simulink model "jplsetispec_thresh_rev003"  (Simulink 6.2)
settings: Solver=ode45  StartTime=0.0  StopTime=100  RelTol=1e-3
libraries: xbsIndex_r3 x776, xps_library x53, casper_library x4
(part 2 of 5)

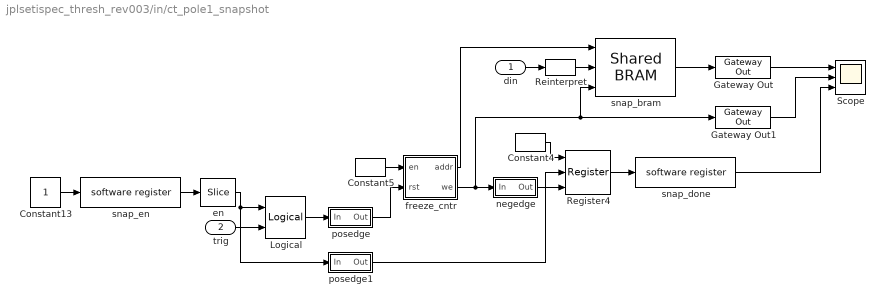
== system jplsetispec_thresh_rev003/in/ct_pole1_snapshot ==
  din : Inport  Port=1  LatchInput=off
  trig : Inport  Port=2  LatchInput=off
  Constant13 : Constant
  Constant4 : xbsIndex_r3/Constant  const=1  equ=P=C  arith_type=Unsigned  n_bits=1  bin_pt=0  opselect=C  inp2=PCIN>>17  opr=+  inp1=P  carry=CIN  iostate=0  explicit_period=on  period=1  dbl_ovrd=off
  Constant5 : xbsIndex_r3/Constant  const=1  equ=P=C  arith_type=Boolean  n_bits=1  bin_pt=0  opselect=C  inp2=PCIN>>17  opr=+  inp1=P  carry=CIN  iostate=0  explicit_period=on  period=1  dbl_ovrd=off
  Gateway Out : xbsIndex_r3/Gateway Out  output_type=Double  nbits=8  bin_pt=6  arith_type=Boolean  quantization=Truncate  overflow=Wrap  hdl_port=off  timing_constraint=None  locs_specified=off  LOCs={}  needs_fixed_name=off  show_param=off
      settings: xl_area=[0, 0, 0, 0, 0, 0, 0]
  Gateway Out1 : xbsIndex_r3/Gateway Out  output_type=Double  nbits=8  bin_pt=6  arith_type=Boolean  quantization=Truncate  overflow=Wrap  hdl_port=off  timing_constraint=None  locs_specified=off  LOCs={}  needs_fixed_name=off  show_param=off
      settings: xl_area=[0, 0, 0, 0, 0, 0, 0]
  Logical : xbsIndex_r3/Logical  logical_function=AND  inputs=2  precision=Full  arith_type=Unsigned  n_bits=8  bin_pt=2  align_bp=on  latency=0  explicit_period=on  period=1  en=off  dbl_ovrd=off  show_param=off
      settings: xl_area=[0, 0, 0, 0, 0, 0, 0]
  Register4 : xbsIndex_r3/Register  init=0  reg_only_valid=off  explicit_period=off  period=1  rst=on  en=on  out_en=off  dbl_ovrd=off  show_param=off
      settings: xl_area=[0, 0, 0, 0, 0, 0, 0]
  Reinterpret : xbsIndex_r3/Reinterpret  force_arith_type=on  arith_type=Unsigned  force_bin_pt=on  bin_pt=0  force_valid=on
  Scope : Scope  NumInputPorts=3
      settings: YMin=-5~-5~-5  YMax=5~5~5
  en : xbsIndex_r3/Slice  mode=Lower Bit Location + Width  nbits=1  bit1=0  base1=LSB of Input  bit0=0  base0=LSB of Input  boolean_output=on  explicit_period=off  period=1  dbl_ovrd=off
  freeze_cntr : Subsystem  mask{CounterBits=nsamples}
      mask prompts: CounterBits "Counter Length (2^?)"
  negedge : Subsystem  Tag=Rising Edge Detector
  posedge : Subsystem  Tag=Rising Edge Detector
  posedge1 : Subsystem  Tag=Rising Edge Detector
  snap_bram : xps_library/Shared BRAM  Tag=xps:bram  arith_type=Unsigned  addr_width=nsamples  data_width=32  data_bin_pt=0  init_vals=0  sample_rate=1
  snap_done : xps_library/software register  Tag=xps:sw_reg  io_dir=To Processor  arith_type=Unsigned  bitwidth=32  bin_pt=0  sample_period=1  gw_name=jplsetispec_thresh_rev003_in_ct_pole1_snapshot_snap_done_user_data_in
  snap_en : xps_library/software register  Tag=xps:sw_reg  io_dir=From Processor  arith_type=Unsigned  bitwidth=32  bin_pt=0  sample_period=1  gw_name=jplsetispec_thresh_rev003_in_ct_pole1_snapshot_snap_en_user_data_out
  wires:
  posedge1/1(Out) -> Register4/2
  snap_done/1 -> Scope/3
  Gateway Out1/1 -> Scope/2
  Gateway Out/1 -> Scope/1
  snap_bram/1 -> Gateway Out/1
  freeze_cntr/1(addr) -> snap_bram/1
  en/1 -> posedge1/1(In), Logical/1
  negedge/1(Out) -> Register4/3
  trig/1 -> Logical/2
  posedge/1(Out) -> freeze_cntr/2(rst)
  Logical/1 -> posedge/1(In)
  freeze_cntr/2(we) -> Gateway Out1/1, snap_bram/3, negedge/1(In)
  Constant5/1 -> freeze_cntr/1(en)
  Constant4/1 -> Register4/1
  Register4/1 -> snap_done/1
  Constant13/1 -> snap_en/1
  Reinterpret/1 -> snap_bram/2
  din/1 -> Reinterpret/1
  snap_en/1 -> en/1

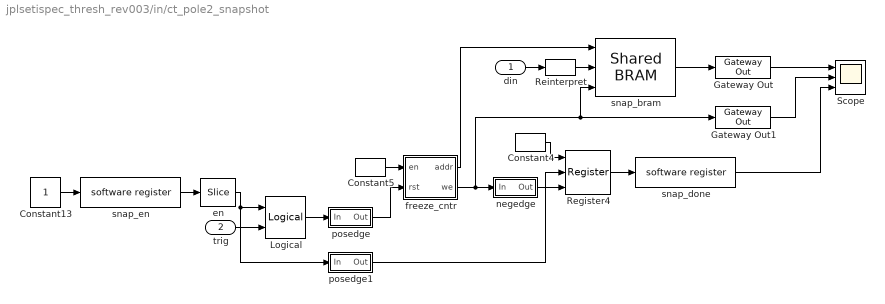
== system jplsetispec_thresh_rev003/in/ct_pole2_snapshot ==
  din : Inport  Port=1  LatchInput=off
  trig : Inport  Port=2  LatchInput=off
  Constant13 : Constant
  Constant4 : xbsIndex_r3/Constant  const=1  equ=P=C  arith_type=Unsigned  n_bits=1  bin_pt=0  opselect=C  inp2=PCIN>>17  opr=+  inp1=P  carry=CIN  iostate=0  explicit_period=on  period=1  dbl_ovrd=off
  Constant5 : xbsIndex_r3/Constant  const=1  equ=P=C  arith_type=Boolean  n_bits=1  bin_pt=0  opselect=C  inp2=PCIN>>17  opr=+  inp1=P  carry=CIN  iostate=0  explicit_period=on  period=1  dbl_ovrd=off
  Gateway Out : xbsIndex_r3/Gateway Out  output_type=Double  nbits=8  bin_pt=6  arith_type=Boolean  quantization=Truncate  overflow=Wrap  hdl_port=off  timing_constraint=None  locs_specified=off  LOCs={}  needs_fixed_name=off  show_param=off
      settings: xl_area=[0, 0, 0, 0, 0, 0, 0]
  Gateway Out1 : xbsIndex_r3/Gateway Out  output_type=Double  nbits=8  bin_pt=6  arith_type=Boolean  quantization=Truncate  overflow=Wrap  hdl_port=off  timing_constraint=None  locs_specified=off  LOCs={}  needs_fixed_name=off  show_param=off
      settings: xl_area=[0, 0, 0, 0, 0, 0, 0]
  Logical : xbsIndex_r3/Logical  logical_function=AND  inputs=2  precision=Full  arith_type=Unsigned  n_bits=8  bin_pt=2  align_bp=on  latency=0  explicit_period=on  period=1  en=off  dbl_ovrd=off  show_param=off
      settings: xl_area=[0, 0, 0, 0, 0, 0, 0]
  Register4 : xbsIndex_r3/Register  init=0  reg_only_valid=off  explicit_period=off  period=1  rst=on  en=on  out_en=off  dbl_ovrd=off  show_param=off
      settings: xl_area=[0, 0, 0, 0, 0, 0, 0]
  Reinterpret : xbsIndex_r3/Reinterpret  force_arith_type=on  arith_type=Unsigned  force_bin_pt=on  bin_pt=0  force_valid=on
  Scope : Scope  NumInputPorts=3
      settings: YMin=-5~-5~-5  YMax=5~5~5
  en : xbsIndex_r3/Slice  mode=Lower Bit Location + Width  nbits=1  bit1=0  base1=LSB of Input  bit0=0  base0=LSB of Input  boolean_output=on  explicit_period=off  period=1  dbl_ovrd=off
  freeze_cntr : Subsystem  mask{CounterBits=nsamples}
      mask prompts: CounterBits "Counter Length (2^?)"
  negedge : Subsystem  Tag=Rising Edge Detector
  posedge : Subsystem  Tag=Rising Edge Detector
  posedge1 : Subsystem  Tag=Rising Edge Detector
  snap_bram : xps_library/Shared BRAM  Tag=xps:bram  arith_type=Unsigned  addr_width=nsamples  data_width=32  data_bin_pt=0  init_vals=0  sample_rate=1
  snap_done : xps_library/software register  Tag=xps:sw_reg  io_dir=To Processor  arith_type=Unsigned  bitwidth=32  bin_pt=0  sample_period=1  gw_name=jplsetispec_thresh_rev003_in_ct_pole2_snapshot_snap_done_user_data_in
  snap_en : xps_library/software register  Tag=xps:sw_reg  io_dir=From Processor  arith_type=Unsigned  bitwidth=32  bin_pt=0  sample_period=1  gw_name=jplsetispec_thresh_rev003_in_ct_pole2_snapshot_snap_en_user_data_out
  wires:
  snap_en/1 -> en/1
  din/1 -> Reinterpret/1
  Reinterpret/1 -> snap_bram/2
  Constant13/1 -> snap_en/1
  Register4/1 -> snap_done/1
  Constant4/1 -> Register4/1
  Constant5/1 -> freeze_cntr/1(en)
  freeze_cntr/2(we) -> negedge/1(In), snap_bram/3, Gateway Out1/1
  Logical/1 -> posedge/1(In)
  posedge/1(Out) -> freeze_cntr/2(rst)
  trig/1 -> Logical/2
  negedge/1(Out) -> Register4/3
  en/1 -> Logical/1, posedge1/1(In)
  freeze_cntr/1(addr) -> snap_bram/1
  snap_bram/1 -> Gateway Out/1
  Gateway Out/1 -> Scope/1
  Gateway Out1/1 -> Scope/2
  snap_done/1 -> Scope/3
  posedge1/1(Out) -> Register4/2

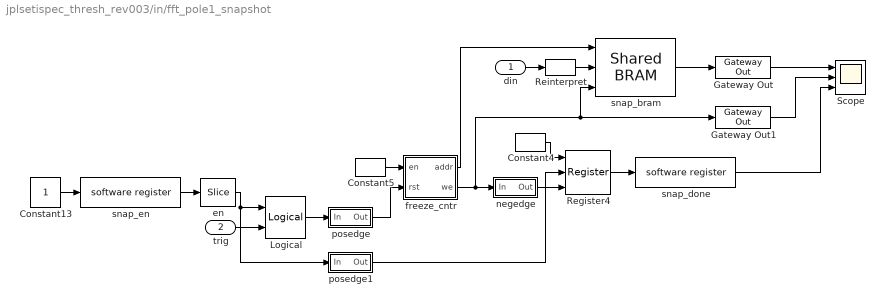
== system jplsetispec_thresh_rev003/in/fft_pole1_snapshot ==
  din : Inport  Port=1  LatchInput=off
  trig : Inport  Port=2  LatchInput=off
  Constant13 : Constant
  Constant4 : xbsIndex_r3/Constant  const=1  equ=P=C  arith_type=Unsigned  n_bits=1  bin_pt=0  opselect=C  inp2=PCIN>>17  opr=+  inp1=P  carry=CIN  iostate=0  explicit_period=on  period=1  dbl_ovrd=off
  Constant5 : xbsIndex_r3/Constant  const=1  equ=P=C  arith_type=Boolean  n_bits=1  bin_pt=0  opselect=C  inp2=PCIN>>17  opr=+  inp1=P  carry=CIN  iostate=0  explicit_period=on  period=1  dbl_ovrd=off
  Gateway Out : xbsIndex_r3/Gateway Out  output_type=Double  nbits=8  bin_pt=6  arith_type=Boolean  quantization=Truncate  overflow=Wrap  hdl_port=off  timing_constraint=None  locs_specified=off  LOCs={}  needs_fixed_name=off  show_param=off
      settings: xl_area=[0, 0, 0, 0, 0, 0, 0]
  Gateway Out1 : xbsIndex_r3/Gateway Out  output_type=Double  nbits=8  bin_pt=6  arith_type=Boolean  quantization=Truncate  overflow=Wrap  hdl_port=off  timing_constraint=None  locs_specified=off  LOCs={}  needs_fixed_name=off  show_param=off
      settings: xl_area=[0, 0, 0, 0, 0, 0, 0]
  Logical : xbsIndex_r3/Logical  logical_function=AND  inputs=2  precision=Full  arith_type=Unsigned  n_bits=8  bin_pt=2  align_bp=on  latency=0  explicit_period=on  period=1  en=off  dbl_ovrd=off  show_param=off
      settings: xl_area=[0, 0, 0, 0, 0, 0, 0]
  Register4 : xbsIndex_r3/Register  init=0  reg_only_valid=off  explicit_period=off  period=1  rst=on  en=on  out_en=off  dbl_ovrd=off  show_param=off
      settings: xl_area=[0, 0, 0, 0, 0, 0, 0]
  Reinterpret : xbsIndex_r3/Reinterpret  force_arith_type=on  arith_type=Unsigned  force_bin_pt=on  bin_pt=0  force_valid=on
  Scope : Scope  NumInputPorts=3
      settings: YMin=-5~-5~-5  YMax=5~5~5
  en : xbsIndex_r3/Slice  mode=Lower Bit Location + Width  nbits=1  bit1=0  base1=LSB of Input  bit0=0  base0=LSB of Input  boolean_output=on  explicit_period=off  period=1  dbl_ovrd=off
  freeze_cntr : Subsystem  mask{CounterBits=nsamples}
      mask prompts: CounterBits "Counter Length (2^?)"
  negedge : Subsystem  Tag=Rising Edge Detector
  posedge : Subsystem  Tag=Rising Edge Detector
  posedge1 : Subsystem  Tag=Rising Edge Detector
  snap_bram : xps_library/Shared BRAM  Tag=xps:bram  arith_type=Unsigned  addr_width=nsamples  data_width=32  data_bin_pt=0  init_vals=0  sample_rate=1
  snap_done : xps_library/software register  Tag=xps:sw_reg  io_dir=To Processor  arith_type=Unsigned  bitwidth=32  bin_pt=0  sample_period=1  gw_name=jplsetispec_thresh_rev003_in_fft_pole1_snapshot_snap_done_user_data_in
  snap_en : xps_library/software register  Tag=xps:sw_reg  io_dir=From Processor  arith_type=Unsigned  bitwidth=32  bin_pt=0  sample_period=1  gw_name=jplsetispec_thresh_rev003_in_fft_pole1_snapshot_snap_en_user_data_out
  wires:
  posedge1/1(Out) -> Register4/2
  snap_done/1 -> Scope/3
  Gateway Out1/1 -> Scope/2
  Gateway Out/1 -> Scope/1
  snap_bram/1 -> Gateway Out/1
  freeze_cntr/1(addr) -> snap_bram/1
  en/1 -> posedge1/1(In), Logical/1
  negedge/1(Out) -> Register4/3
  trig/1 -> Logical/2
  posedge/1(Out) -> freeze_cntr/2(rst)
  Logical/1 -> posedge/1(In)
  freeze_cntr/2(we) -> Gateway Out1/1, snap_bram/3, negedge/1(In)
  Constant5/1 -> freeze_cntr/1(en)
  Constant4/1 -> Register4/1
  Register4/1 -> snap_done/1
  Constant13/1 -> snap_en/1
  Reinterpret/1 -> snap_bram/2
  din/1 -> Reinterpret/1
  snap_en/1 -> en/1

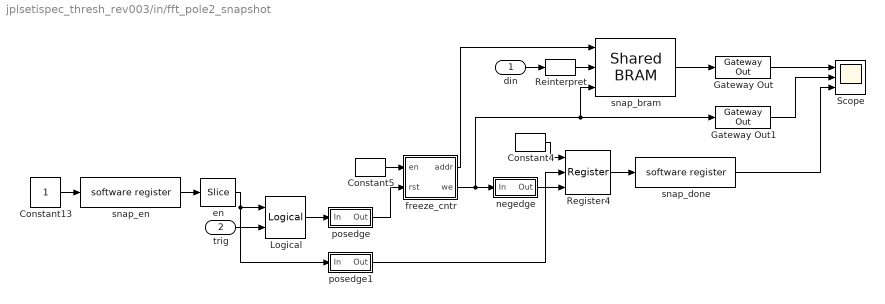
== system jplsetispec_thresh_rev003/in/fft_pole2_snapshot ==
  din : Inport  Port=1  LatchInput=off
  trig : Inport  Port=2  LatchInput=off
  Constant13 : Constant
  Constant4 : xbsIndex_r3/Constant  const=1  equ=P=C  arith_type=Unsigned  n_bits=1  bin_pt=0  opselect=C  inp2=PCIN>>17  opr=+  inp1=P  carry=CIN  iostate=0  explicit_period=on  period=1  dbl_ovrd=off
  Constant5 : xbsIndex_r3/Constant  const=1  equ=P=C  arith_type=Boolean  n_bits=1  bin_pt=0  opselect=C  inp2=PCIN>>17  opr=+  inp1=P  carry=CIN  iostate=0  explicit_period=on  period=1  dbl_ovrd=off
  Gateway Out : xbsIndex_r3/Gateway Out  output_type=Double  nbits=8  bin_pt=6  arith_type=Boolean  quantization=Truncate  overflow=Wrap  hdl_port=off  timing_constraint=None  locs_specified=off  LOCs={}  needs_fixed_name=off  show_param=off
      settings: xl_area=[0, 0, 0, 0, 0, 0, 0]
  Gateway Out1 : xbsIndex_r3/Gateway Out  output_type=Double  nbits=8  bin_pt=6  arith_type=Boolean  quantization=Truncate  overflow=Wrap  hdl_port=off  timing_constraint=None  locs_specified=off  LOCs={}  needs_fixed_name=off  show_param=off
      settings: xl_area=[0, 0, 0, 0, 0, 0, 0]
  Logical : xbsIndex_r3/Logical  logical_function=AND  inputs=2  precision=Full  arith_type=Unsigned  n_bits=8  bin_pt=2  align_bp=on  latency=0  explicit_period=on  period=1  en=off  dbl_ovrd=off  show_param=off
      settings: xl_area=[0, 0, 0, 0, 0, 0, 0]
  Register4 : xbsIndex_r3/Register  init=0  reg_only_valid=off  explicit_period=off  period=1  rst=on  en=on  out_en=off  dbl_ovrd=off  show_param=off
      settings: xl_area=[0, 0, 0, 0, 0, 0, 0]
  Reinterpret : xbsIndex_r3/Reinterpret  force_arith_type=on  arith_type=Unsigned  force_bin_pt=on  bin_pt=0  force_valid=on
  Scope : Scope  NumInputPorts=3
      settings: YMin=-5~-5~-5  YMax=5~5~5
  en : xbsIndex_r3/Slice  mode=Lower Bit Location + Width  nbits=1  bit1=0  base1=LSB of Input  bit0=0  base0=LSB of Input  boolean_output=on  explicit_period=off  period=1  dbl_ovrd=off
  freeze_cntr : Subsystem  mask{CounterBits=nsamples}
      mask prompts: CounterBits "Counter Length (2^?)"
  negedge : Subsystem  Tag=Rising Edge Detector
  posedge : Subsystem  Tag=Rising Edge Detector
  posedge1 : Subsystem  Tag=Rising Edge Detector
  snap_bram : xps_library/Shared BRAM  Tag=xps:bram  arith_type=Unsigned  addr_width=nsamples  data_width=32  data_bin_pt=0  init_vals=0  sample_rate=1
  snap_done : xps_library/software register  Tag=xps:sw_reg  io_dir=To Processor  arith_type=Unsigned  bitwidth=32  bin_pt=0  sample_period=1  gw_name=jplsetispec_thresh_rev003_in_fft_pole2_snapshot_snap_done_user_data_in
  snap_en : xps_library/software register  Tag=xps:sw_reg  io_dir=From Processor  arith_type=Unsigned  bitwidth=32  bin_pt=0  sample_period=1  gw_name=jplsetispec_thresh_rev003_in_fft_pole2_snapshot_snap_en_user_data_out
  wires:
  snap_en/1 -> en/1
  din/1 -> Reinterpret/1
  Reinterpret/1 -> snap_bram/2
  Constant13/1 -> snap_en/1
  Register4/1 -> snap_done/1
  Constant4/1 -> Register4/1
  Constant5/1 -> freeze_cntr/1(en)
  freeze_cntr/2(we) -> negedge/1(In), snap_bram/3, Gateway Out1/1
  Logical/1 -> posedge/1(In)
  posedge/1(Out) -> freeze_cntr/2(rst)
  trig/1 -> Logical/2
  negedge/1(Out) -> Register4/3
  en/1 -> Logical/1, posedge1/1(In)
  freeze_cntr/1(addr) -> snap_bram/1
  snap_bram/1 -> Gateway Out/1
  Gateway Out/1 -> Scope/1
  Gateway Out1/1 -> Scope/2
  snap_done/1 -> Scope/3
  posedge1/1(Out) -> Register4/2

== system jplsetispec_thresh_rev003/in/posedge ==
  in : Inport  Port=1  LatchInput=off
  Delay : xbsIndex_r3/Delay  latency=1  reg_retiming=off  explicit_period=off  period=1  en=off  accept_only_valid=off  init_zero=on  dbl_ovrd=off  show_param=off
      settings: xl_area=[0, 0, 0, 0, 0, 0, 0]
  Inverter : xbsIndex_r3/Inverter  latency=0  explicit_period=off  period=1  en=off  dbl_ovrd=off  show_param=off
      settings: xl_area=[0, 0, 0, 0, 0, 0, 0]
  Logical : xbsIndex_r3/Logical  logical_function=AND  inputs=2  precision=Full  arith_type=Unsigned  n_bits=8  bin_pt=2  align_bp=on  latency=0  explicit_period=off  period=1  en=off  dbl_ovrd=off  show_param=off
      settings: xl_area=[0, 0, 0, 0, 0, 0, 0]
  detect : Outport
  wires:
  Logical/1 -> detect/1
  in/1 -> Logical/2, Delay/1
  Inverter/1 -> Logical/1
  Delay/1 -> Inverter/1

== system jplsetispec_thresh_rev003/in/posedge1 ==
  in : Inport  Port=1  LatchInput=off
  Delay : xbsIndex_r3/Delay  latency=1  reg_retiming=off  explicit_period=off  period=1  en=off  accept_only_valid=off  init_zero=on  dbl_ovrd=off  show_param=off
      settings: xl_area=[0, 0, 0, 0, 0, 0, 0]
  Inverter : xbsIndex_r3/Inverter  latency=0  explicit_period=off  period=1  en=off  dbl_ovrd=off  show_param=off
      settings: xl_area=[0, 0, 0, 0, 0, 0, 0]
  Logical : xbsIndex_r3/Logical  logical_function=AND  inputs=2  precision=Full  arith_type=Unsigned  n_bits=8  bin_pt=2  align_bp=on  latency=0  explicit_period=off  period=1  en=off  dbl_ovrd=off  show_param=off
      settings: xl_area=[0, 0, 0, 0, 0, 0, 0]
  detect : Outport
  wires:
  Delay/1 -> Inverter/1
  Inverter/1 -> Logical/1
  in/1 -> Delay/1, Logical/2
  Logical/1 -> detect/1

== system jplsetispec_thresh_rev003/in/posedge2 ==
  in : Inport  Port=1  LatchInput=off
  Delay : xbsIndex_r3/Delay  latency=1  reg_retiming=off  explicit_period=off  period=1  en=off  accept_only_valid=off  init_zero=on  dbl_ovrd=off  show_param=off
      settings: xl_area=[0, 0, 0, 0, 0, 0, 0]
  Inverter : xbsIndex_r3/Inverter  latency=0  explicit_period=off  period=1  en=off  dbl_ovrd=off  show_param=off
      settings: xl_area=[0, 0, 0, 0, 0, 0, 0]
  Logical : xbsIndex_r3/Logical  logical_function=AND  inputs=2  precision=Full  arith_type=Unsigned  n_bits=8  bin_pt=2  align_bp=on  latency=0  explicit_period=off  period=1  en=off  dbl_ovrd=off  show_param=off
      settings: xl_area=[0, 0, 0, 0, 0, 0, 0]
  detect : Outport
  wires:
  Delay/1 -> Inverter/1
  Inverter/1 -> Logical/1
  in/1 -> Delay/1, Logical/2
  Logical/1 -> detect/1

== system jplsetispec_thresh_rev003/in/posedge3 ==
  in : Inport  Port=1  LatchInput=off
  Delay : xbsIndex_r3/Delay  latency=1  reg_retiming=off  explicit_period=off  period=1  en=off  accept_only_valid=off  init_zero=on  dbl_ovrd=off  show_param=off
      settings: xl_area=[0, 0, 0, 0, 0, 0, 0]
  Inverter : xbsIndex_r3/Inverter  latency=0  explicit_period=off  period=1  en=off  dbl_ovrd=off  show_param=off
      settings: xl_area=[0, 0, 0, 0, 0, 0, 0]
  Logical : xbsIndex_r3/Logical  logical_function=AND  inputs=2  precision=Full  arith_type=Unsigned  n_bits=8  bin_pt=2  align_bp=on  latency=0  explicit_period=off  period=1  en=off  dbl_ovrd=off  show_param=off
      settings: xl_area=[0, 0, 0, 0, 0, 0, 0]
  detect : Outport
  wires:
  Logical/1 -> detect/1
  in/1 -> Logical/2, Delay/1
  Inverter/1 -> Logical/1
  Delay/1 -> Inverter/1

== system jplsetispec_thresh_rev003/in/posedge4 ==
  in : Inport  Port=1  LatchInput=off
  Delay : xbsIndex_r3/Delay  latency=1  reg_retiming=off  explicit_period=off  period=1  en=off  accept_only_valid=off  init_zero=on  dbl_ovrd=off  show_param=off
      settings: xl_area=[0, 0, 0, 0, 0, 0, 0]
  Inverter : xbsIndex_r3/Inverter  latency=0  explicit_period=off  period=1  en=off  dbl_ovrd=off  show_param=off
      settings: xl_area=[0, 0, 0, 0, 0, 0, 0]
  Logical : xbsIndex_r3/Logical  logical_function=AND  inputs=2  precision=Full  arith_type=Unsigned  n_bits=8  bin_pt=2  align_bp=on  latency=0  explicit_period=off  period=1  en=off  dbl_ovrd=off  show_param=off
      settings: xl_area=[0, 0, 0, 0, 0, 0, 0]
  detect : Outport
  wires:
  Delay/1 -> Inverter/1
  Inverter/1 -> Logical/1
  in/1 -> Delay/1, Logical/2
  Logical/1 -> detect/1

== system jplsetispec_thresh_rev003/in/posedge5 ==
  in : Inport  Port=1  LatchInput=off
  Delay : xbsIndex_r3/Delay  latency=1  reg_retiming=off  explicit_period=off  period=1  en=off  accept_only_valid=off  init_zero=on  dbl_ovrd=off  show_param=off
      settings: xl_area=[0, 0, 0, 0, 0, 0, 0]
  Inverter : xbsIndex_r3/Inverter  latency=0  explicit_period=off  period=1  en=off  dbl_ovrd=off  show_param=off
      settings: xl_area=[0, 0, 0, 0, 0, 0, 0]
  Logical : xbsIndex_r3/Logical  logical_function=AND  inputs=2  precision=Full  arith_type=Unsigned  n_bits=8  bin_pt=2  align_bp=on  latency=0  explicit_period=off  period=1  en=off  dbl_ovrd=off  show_param=off
      settings: xl_area=[0, 0, 0, 0, 0, 0, 0]
  detect : Outport
  wires:
  Logical/1 -> detect/1
  in/1 -> Logical/2, Delay/1
  Inverter/1 -> Logical/1
  Delay/1 -> Inverter/1

== system jplsetispec_thresh_rev003/in/pulse_extender ==
  in : Inport  Port=1  LatchInput=off
  Constant : xbsIndex_r3/Constant  const=1  equ=P=C  arith_type=Boolean  n_bits=1  bin_pt=0  opselect=C  inp2=PCIN>>17  opr=+  inp1=P  carry=CIN  iostate=0  explicit_period=off  period=1  dbl_ovrd=off
  Constant17 : xbsIndex_r3/Constant  const=pulse_len  equ=P=C  arith_type=Unsigned  n_bits=bits  bin_pt=0  opselect=C  inp2=PCIN>>17  opr=+  inp1=P  carry=CIN  iostate=0  explicit_period=on  period=1  dbl_ovrd=off
  Logical : xbsIndex_r3/Logical  logical_function=AND  inputs=2  precision=Full  arith_type=Unsigned  n_bits=8  bin_pt=2  align_bp=on  latency=0  explicit_period=off  period=1  en=off  dbl_ovrd=off  show_param=off
      settings: xl_area=[0, 0, 0, 0, 0, 0, 0]
  Register : xbsIndex_r3/Register  init=0  reg_only_valid=off  explicit_period=off  period=1  rst=off  en=on  out_en=off  dbl_ovrd=off  show_param=off
      settings: xl_area=[0, 0, 0, 0, 0, 0, 0]
  Relational1 : xbsIndex_r3/Relational  mode=a<b  latency=0  explicit_period=off  period=1  en=off  dbl_ovrd=off  show_param=off
      settings: xl_area=[0, 0, 0, 0, 0, 0, 0]
  Terminator : Terminator
  freeze_cntr : Subsystem  mask{CounterBits=bits}
      mask prompts: CounterBits "Counter Length (2^?)"
  posedge : Subsystem  Tag=Rising Edge Detector
  out : Outport
  wires:
  Logical/1 -> out/1
  Register/1 -> Logical/2
  Relational1/1 -> Logical/1
  in/1 -> Register/2, posedge/1(In)
  Constant17/1 -> Relational1/2
  posedge/1(Out) -> freeze_cntr/2(rst)
  freeze_cntr/1(addr) -> Relational1/1
  freeze_cntr/2(we) -> Terminator/1
  Constant/1 -> Register/1, freeze_cntr/1(en)

== system jplsetispec_thresh_rev003/in/pulse_extender1 ==
  in : Inport  Port=1  LatchInput=off
  Constant : xbsIndex_r3/Constant  const=1  equ=P=C  arith_type=Boolean  n_bits=1  bin_pt=0  opselect=C  inp2=PCIN>>17  opr=+  inp1=P  carry=CIN  iostate=0  explicit_period=off  period=1  dbl_ovrd=off
  Constant17 : xbsIndex_r3/Constant  const=pulse_len  equ=P=C  arith_type=Unsigned  n_bits=bits  bin_pt=0  opselect=C  inp2=PCIN>>17  opr=+  inp1=P  carry=CIN  iostate=0  explicit_period=on  period=1  dbl_ovrd=off
  Logical : xbsIndex_r3/Logical  logical_function=AND  inputs=2  precision=Full  arith_type=Unsigned  n_bits=8  bin_pt=2  align_bp=on  latency=0  explicit_period=off  period=1  en=off  dbl_ovrd=off  show_param=off
      settings: xl_area=[0, 0, 0, 0, 0, 0, 0]
  Register : xbsIndex_r3/Register  init=0  reg_only_valid=off  explicit_period=off  period=1  rst=off  en=on  out_en=off  dbl_ovrd=off  show_param=off
      settings: xl_area=[0, 0, 0, 0, 0, 0, 0]
  Relational1 : xbsIndex_r3/Relational  mode=a<b  latency=0  explicit_period=off  period=1  en=off  dbl_ovrd=off  show_param=off
      settings: xl_area=[0, 0, 0, 0, 0, 0, 0]
  Terminator : Terminator
  freeze_cntr : Subsystem  mask{CounterBits=bits}
      mask prompts: CounterBits "Counter Length (2^?)"
  posedge : Subsystem  Tag=Rising Edge Detector
  out : Outport
  wires:
  Logical/1 -> out/1
  Register/1 -> Logical/2
  Relational1/1 -> Logical/1
  in/1 -> Register/2, posedge/1(In)
  Constant17/1 -> Relational1/2
  posedge/1(Out) -> freeze_cntr/2(rst)
  freeze_cntr/1(addr) -> Relational1/1
  freeze_cntr/2(we) -> Terminator/1
  Constant/1 -> Register/1, freeze_cntr/1(en)

== system jplsetispec_thresh_rev003/in/sync_gen ==
  Counter : xbsIndex_r3/Counter  Orientation=left  cnt_type=Free Running  n_bits=syncPeriodBits  bin_pt=0  arith_type=Unsigned  start_count=0  cnt_to=Inf  cnt_by_val=1  operation=Up  explicit_period=off  period=1  load_pin=off  rst=on  en=off  dbl_ovrd=off  show_param=off  use_rpm=on  gen_core=off
      settings: xl_area=[0, 0, 0, 0, 0, 0, 0]
  Relational : xbsIndex_r3/Relational  mode=a=b  latency=1  explicit_period=on  period=1  en=off  dbl_ovrd=off  show_param=off
      settings: xl_area=[0, 0, 0, 0, 0, 0, 0]
  sub_wrap_delay : xbsIndex_r3/AddSub  mode=Subtraction  precision=Full  arith_type=Unsigned  n_bits=8  bin_pt=2  quantization=Truncate  overflow=Wrap  latency=2  explicit_period=off  period=1  use_carryin=off  use_carryout=off  en=off  dbl_ovrd=off  show_param=off  use_core=on  pipeline=off  use_rpm=on  gen_core=off
      settings: xl_area=[0, 0, 0, 0, 0, 0, 0]
  sync_period : xbsIndex_r3/Constant  const=syncPeriod  equ=P=C  arith_type=Unsigned  n_bits=syncPeriodBits  bin_pt=0  opselect=C  inp2=PCIN>>17  opr=+  inp1=P  carry=CIN  iostate=0  explicit_period=on  period=1  dbl_ovrd=off
  wrap_offset : xbsIndex_r3/Constant  const=2  equ=P=C  arith_type=Unsigned  n_bits=syncPeriodBits  bin_pt=0  opselect=C  inp2=PCIN>>17  opr=+  inp1=P  carry=CIN  iostate=0  explicit_period=on  period=1  dbl_ovrd=off
  sync_out : Outport
  wires:
  sub_wrap_delay/1 -> Relational/2
  Relational/1 -> sync_out/1, Counter/1
  Counter/1 -> Relational/1
  sync_period/1 -> sub_wrap_delay/1
  wrap_offset/1 -> sub_wrap_delay/2

== system jplsetispec_thresh_rev003/in/sync_gen1 ==
  Counter : xbsIndex_r3/Counter  Orientation=left  cnt_type=Free Running  n_bits=syncPeriodBits  bin_pt=0  arith_type=Unsigned  start_count=0  cnt_to=Inf  cnt_by_val=1  operation=Up  explicit_period=off  period=1  load_pin=off  rst=on  en=off  dbl_ovrd=off  show_param=off  use_rpm=on  gen_core=off
      settings: xl_area=[0, 0, 0, 0, 0, 0, 0]
  Relational : xbsIndex_r3/Relational  mode=a=b  latency=1  explicit_period=on  period=1  en=off  dbl_ovrd=off  show_param=off
      settings: xl_area=[0, 0, 0, 0, 0, 0, 0]
  sub_wrap_delay : xbsIndex_r3/AddSub  mode=Subtraction  precision=Full  arith_type=Unsigned  n_bits=8  bin_pt=2  quantization=Truncate  overflow=Wrap  latency=2  explicit_period=off  period=1  use_carryin=off  use_carryout=off  en=off  dbl_ovrd=off  show_param=off  use_core=on  pipeline=off  use_rpm=on  gen_core=off
      settings: xl_area=[0, 0, 0, 0, 0, 0, 0]
  sync_period : xbsIndex_r3/Constant  const=syncPeriod  equ=P=C  arith_type=Unsigned  n_bits=syncPeriodBits  bin_pt=0  opselect=C  inp2=PCIN>>17  opr=+  inp1=P  carry=CIN  iostate=0  explicit_period=on  period=1  dbl_ovrd=off
  wrap_offset : xbsIndex_r3/Constant  const=2  equ=P=C  arith_type=Unsigned  n_bits=syncPeriodBits  bin_pt=0  opselect=C  inp2=PCIN>>17  opr=+  inp1=P  carry=CIN  iostate=0  explicit_period=on  period=1  dbl_ovrd=off
  sync_out : Outport
  wires:
  wrap_offset/1 -> sub_wrap_delay/2
  sync_period/1 -> sub_wrap_delay/1
  Counter/1 -> Relational/1
  Relational/1 -> Counter/1, sync_out/1
  sub_wrap_delay/1 -> Relational/2

== system jplsetispec_thresh_rev003/in/tvg ==
  sync : Inport  Port=1  LatchInput=off
  pulse_extender : Subsystem  mask{pulse_len=(2^dataWidth)-1}
      mask prompts: pulse_len "Length of Pulse"
      mask init:
      | bits = 1 + floor(log2(pulse_len));
  tvg_cnt : xbsIndex_r3/Counter  cnt_type=Free Running  n_bits=dataWidth  bin_pt=0  arith_type=Unsigned  start_count=0  cnt_to=2^dataWidth  cnt_by_val=1  operation=Up  explicit_period=off  period=1  load_pin=off  rst=on  en=on  dbl_ovrd=off  show_param=off  use_rpm=on  gen_core=off
      settings: xl_area=[0, 0, 0, 0, 0, 0, 0]
  out : Outport
  wires:
  pulse_extender/1(out) -> tvg_cnt/2
  sync/1 -> pulse_extender/1(in), tvg_cnt/1
  tvg_cnt/1 -> out/1

== system jplsetispec_thresh_rev003/in/tvg1 ==
  sync : Inport  Port=1  LatchInput=off
  pulse_extender : Subsystem  mask{pulse_len=(2^dataWidth)-1}
      mask prompts: pulse_len "Length of Pulse"
      mask init:
      | bits = 1 + floor(log2(pulse_len));
  tvg_cnt : xbsIndex_r3/Counter  cnt_type=Free Running  n_bits=dataWidth  bin_pt=0  arith_type=Unsigned  start_count=0  cnt_to=2^dataWidth  cnt_by_val=1  operation=Up  explicit_period=off  period=1  load_pin=off  rst=on  en=on  dbl_ovrd=off  show_param=off  use_rpm=on  gen_core=off
      settings: xl_area=[0, 0, 0, 0, 0, 0, 0]
  out : Outport
  wires:
  tvg_cnt/1 -> out/1
  sync/1 -> tvg_cnt/1, pulse_extender/1(in)
  pulse_extender/1(out) -> tvg_cnt/2

== system jplsetispec_thresh_rev003/in/tvg2 ==
  sync : Inport  Port=1  LatchInput=off
  pulse_extender : Subsystem  mask{pulse_len=(2^dataWidth)-1}
      mask prompts: pulse_len "Length of Pulse"
      mask init:
      | bits = 1 + floor(log2(pulse_len));
  tvg_cnt : xbsIndex_r3/Counter  cnt_type=Free Running  n_bits=dataWidth  bin_pt=0  arith_type=Unsigned  start_count=0  cnt_to=2^dataWidth  cnt_by_val=1  operation=Up  explicit_period=off  period=1  load_pin=off  rst=on  en=on  dbl_ovrd=off  show_param=off  use_rpm=on  gen_core=off
      settings: xl_area=[0, 0, 0, 0, 0, 0, 0]
  out : Outport
  wires:
  tvg_cnt/1 -> out/1
  sync/1 -> tvg_cnt/1, pulse_extender/1(in)
  pulse_extender/1(out) -> tvg_cnt/2

== system jplsetispec_thresh_rev003/in/tvg3 ==
  sync : Inport  Port=1  LatchInput=off
  pulse_extender : Subsystem  mask{pulse_len=(2^dataWidth)-1}
      mask prompts: pulse_len "Length of Pulse"
      mask init:
      | bits = 1 + floor(log2(pulse_len));
  tvg_cnt : xbsIndex_r3/Counter  cnt_type=Free Running  n_bits=dataWidth  bin_pt=0  arith_type=Unsigned  start_count=0  cnt_to=2^dataWidth  cnt_by_val=1  operation=Up  explicit_period=off  period=1  load_pin=off  rst=on  en=on  dbl_ovrd=off  show_param=off  use_rpm=on  gen_core=off
      settings: xl_area=[0, 0, 0, 0, 0, 0, 0]
  out : Outport
  wires:
  pulse_extender/1(out) -> tvg_cnt/2
  sync/1 -> pulse_extender/1(in), tvg_cnt/1
  tvg_cnt/1 -> out/1

== system jplsetispec_thresh_rev003/rec/LED_fifo1we ==
  Sync_In : Inport  Port=1  LatchInput=off
  Scope : Scope
  gpio : xps_library/gpio  Tag=xps:gpio  io_group=BEE2_usr:led  io_dir=out  arith_type=Boolean  bitwidth=1  bin_pt=0  bit_index=4  sample_period=1  use_single_ended=off  use_ddr=off  reg_iob=on  reg_clk_phase=0  termination=None
  wires:
  gpio/1 -> Scope/1
  Sync_In/1 -> gpio/1

== system jplsetispec_thresh_rev003/rec/LED_fifo2we ==
  Sync_In : Inport  Port=1  LatchInput=off
  Scope : Scope
  gpio : xps_library/gpio  Tag=xps:gpio  io_group=BEE2_usr:led  io_dir=out  arith_type=Boolean  bitwidth=1  bin_pt=0  bit_index=5  sample_period=1  use_single_ended=off  use_ddr=off  reg_iob=on  reg_clk_phase=0  termination=None
  wires:
  gpio/1 -> Scope/1
  Sync_In/1 -> gpio/1

== system jplsetispec_thresh_rev003/rec/reg_once ==
  d : Inport  Port=1  LatchInput=off
  en : Inport  Port=2  LatchInput=off
  Convert : xbsIndex_r3/Convert  arith_type=Boolean  n_bits=8  bin_pt=6  quantization=Truncate  overflow=Wrap  latency=0  explicit_period=off  period=1  dbl_ovrd=off  show_param=off  inserted_by_tool=off  pipeline=off
      settings: xl_area=[0, 0, 0, 0, 0, 0, 0]
  Convert1 : xbsIndex_r3/Convert  arith_type=Boolean  n_bits=8  bin_pt=6  quantization=Truncate  overflow=Wrap  latency=0  explicit_period=off  period=1  dbl_ovrd=off  show_param=off  inserted_by_tool=off  pipeline=off
      settings: xl_area=[0, 0, 0, 0, 0, 0, 0]
  Register1 : xbsIndex_r3/Register  init=0  reg_only_valid=off  explicit_period=on  period=1  rst=off  en=on  out_en=off  dbl_ovrd=off  show_param=off
      settings: xl_area=[0, 0, 0, 0, 0, 0, 0]
  Register23 : xbsIndex_r3/Register  init=0  reg_only_valid=off  explicit_period=on  period=1  rst=off  en=on  out_en=off  dbl_ovrd=off  show_param=off
      settings: xl_area=[0, 0, 0, 0, 0, 0, 0]
  edge1 : xbsIndex_r3/Expression  expression=a & ~b  precision=Full  arith_type=Unsigned  n_bits=8  bin_pt=2  align_bp=on  latency=0  explicit_period=off  period=1  en=off  dbl_ovrd=off  show_param=off
      settings: xl_area=[0, 0, 0, 0, 0, 0, 0]
  q : Outport
  wires:
  Convert1/1 -> edge1/1, Register1/1, Register1/2
  Convert/1 -> Register23/2
  Register1/1 -> edge1/2
  en/1 -> Convert1/1
  edge1/1 -> Convert/1
  d/1 -> Register23/1
  Register23/1 -> q/1

== system jplsetispec_thresh_rev003/rec/reg_once1 ==
  d : Inport  Port=1  LatchInput=off
  en : Inport  Port=2  LatchInput=off
  Convert : xbsIndex_r3/Convert  arith_type=Boolean  n_bits=8  bin_pt=6  quantization=Truncate  overflow=Wrap  latency=0  explicit_period=off  period=1  dbl_ovrd=off  show_param=off  inserted_by_tool=off  pipeline=off
      settings: xl_area=[0, 0, 0, 0, 0, 0, 0]
  Convert1 : xbsIndex_r3/Convert  arith_type=Boolean  n_bits=8  bin_pt=6  quantization=Truncate  overflow=Wrap  latency=0  explicit_period=off  period=1  dbl_ovrd=off  show_param=off  inserted_by_tool=off  pipeline=off
      settings: xl_area=[0, 0, 0, 0, 0, 0, 0]
  Register1 : xbsIndex_r3/Register  init=0  reg_only_valid=off  explicit_period=on  period=1  rst=off  en=on  out_en=off  dbl_ovrd=off  show_param=off
      settings: xl_area=[0, 0, 0, 0, 0, 0, 0]
  Register23 : xbsIndex_r3/Register  init=0  reg_only_valid=off  explicit_period=on  period=1  rst=off  en=on  out_en=off  dbl_ovrd=off  show_param=off
      settings: xl_area=[0, 0, 0, 0, 0, 0, 0]
  edge1 : xbsIndex_r3/Expression  expression=a & ~b  precision=Full  arith_type=Unsigned  n_bits=8  bin_pt=2  align_bp=on  latency=0  explicit_period=off  period=1  en=off  dbl_ovrd=off  show_param=off
      settings: xl_area=[0, 0, 0, 0, 0, 0, 0]
  q : Outport
  wires:
  Register23/1 -> q/1
  d/1 -> Register23/1
  edge1/1 -> Convert/1
  en/1 -> Convert1/1
  Register1/1 -> edge1/2
  Convert/1 -> Register23/2
  Convert1/1 -> Register1/2, Register1/1, edge1/1

== system jplsetispec_thresh_rev003/rec/reg_once2 ==
  d : Inport  Port=1  LatchInput=off
  en : Inport  Port=2  LatchInput=off
  Convert : xbsIndex_r3/Convert  arith_type=Boolean  n_bits=8  bin_pt=6  quantization=Truncate  overflow=Wrap  latency=0  explicit_period=off  period=1  dbl_ovrd=off  show_param=off  inserted_by_tool=off  pipeline=off
      settings: xl_area=[0, 0, 0, 0, 0, 0, 0]
  Convert1 : xbsIndex_r3/Convert  arith_type=Boolean  n_bits=8  bin_pt=6  quantization=Truncate  overflow=Wrap  latency=0  explicit_period=off  period=1  dbl_ovrd=off  show_param=off  inserted_by_tool=off  pipeline=off
      settings: xl_area=[0, 0, 0, 0, 0, 0, 0]
  Register1 : xbsIndex_r3/Register  init=0  reg_only_valid=off  explicit_period=on  period=1  rst=off  en=on  out_en=off  dbl_ovrd=off  show_param=off
      settings: xl_area=[0, 0, 0, 0, 0, 0, 0]
  Register23 : xbsIndex_r3/Register  init=0  reg_only_valid=off  explicit_period=on  period=1  rst=off  en=on  out_en=off  dbl_ovrd=off  show_param=off
      settings: xl_area=[0, 0, 0, 0, 0, 0, 0]
  edge1 : xbsIndex_r3/Expression  expression=a & ~b  precision=Full  arith_type=Unsigned  n_bits=8  bin_pt=2  align_bp=on  latency=0  explicit_period=off  period=1  en=off  dbl_ovrd=off  show_param=off
      settings: xl_area=[0, 0, 0, 0, 0, 0, 0]
  q : Outport
  wires:
  Convert1/1 -> edge1/1, Register1/1, Register1/2
  Convert/1 -> Register23/2
  Register1/1 -> edge1/2
  en/1 -> Convert1/1
  edge1/1 -> Convert/1
  d/1 -> Register23/1
  Register23/1 -> q/1

== system jplsetispec_thresh_rev003/rec/reg_once3 ==
  d : Inport  Port=1  LatchInput=off
  en : Inport  Port=2  LatchInput=off
  Convert : xbsIndex_r3/Convert  arith_type=Boolean  n_bits=8  bin_pt=6  quantization=Truncate  overflow=Wrap  latency=0  explicit_period=off  period=1  dbl_ovrd=off  show_param=off  inserted_by_tool=off  pipeline=off
      settings: xl_area=[0, 0, 0, 0, 0, 0, 0]
  Convert1 : xbsIndex_r3/Convert  arith_type=Boolean  n_bits=8  bin_pt=6  quantization=Truncate  overflow=Wrap  latency=0  explicit_period=off  period=1  dbl_ovrd=off  show_param=off  inserted_by_tool=off  pipeline=off
      settings: xl_area=[0, 0, 0, 0, 0, 0, 0]
  Register1 : xbsIndex_r3/Register  init=0  reg_only_valid=off  explicit_period=on  period=1  rst=off  en=on  out_en=off  dbl_ovrd=off  show_param=off
      settings: xl_area=[0, 0, 0, 0, 0, 0, 0]
  Register23 : xbsIndex_r3/Register  init=0  reg_only_valid=off  explicit_period=on  period=1  rst=off  en=on  out_en=off  dbl_ovrd=off  show_param=off
      settings: xl_area=[0, 0, 0, 0, 0, 0, 0]
  edge1 : xbsIndex_r3/Expression  expression=a & ~b  precision=Full  arith_type=Unsigned  n_bits=8  bin_pt=2  align_bp=on  latency=0  explicit_period=off  period=1  en=off  dbl_ovrd=off  show_param=off
      settings: xl_area=[0, 0, 0, 0, 0, 0, 0]
  q : Outport
  wires:
  Register23/1 -> q/1
  d/1 -> Register23/1
  edge1/1 -> Convert/1
  en/1 -> Convert1/1
  Register1/1 -> edge1/2
  Convert/1 -> Register23/2
  Convert1/1 -> Register1/2, Register1/1, edge1/1

== system jplsetispec_thresh_rev003/thr/LED_p1event ==
  Sync_In : Inport  Port=1  LatchInput=off
  Scope : Scope
  gpio : xps_library/gpio  Tag=xps:gpio  io_group=BEE2_usr:led  io_dir=out  arith_type=Boolean  bitwidth=1  bin_pt=0  bit_index=2  sample_period=1  use_single_ended=off  use_ddr=off  reg_iob=on  reg_clk_phase=0  termination=None
  wires:
  gpio/1 -> Scope/1
  Sync_In/1 -> gpio/1

== system jplsetispec_thresh_rev003/thr/LED_p2event ==
  Sync_In : Inport  Port=1  LatchInput=off
  Scope : Scope
  gpio : xps_library/gpio  Tag=xps:gpio  io_group=BEE2_usr:led  io_dir=out  arith_type=Boolean  bitwidth=1  bin_pt=0  bit_index=3  sample_period=1  use_single_ended=off  use_ddr=off  reg_iob=on  reg_clk_phase=0  termination=None
  wires:
  Sync_In/1 -> gpio/1
  gpio/1 -> Scope/1

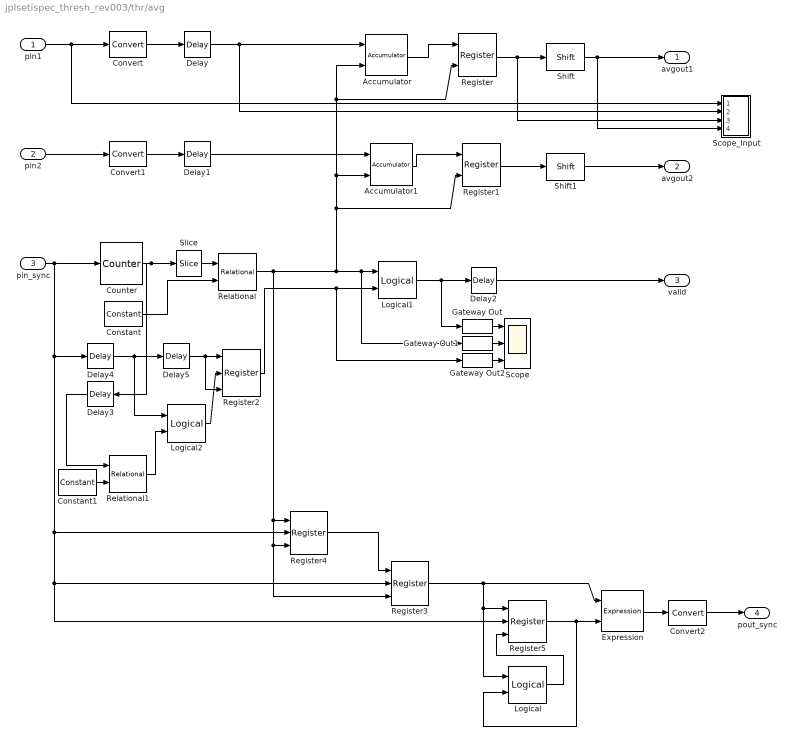
== system jplsetispec_thresh_rev003/thr/avg ==
  pin1 : Inport  Port=1  LatchInput=off
  pin2 : Inport  Port=2  LatchInput=off
  pin_sync : Inport  Port=3  LatchInput=off
  Accumulator : xbsIndex_r3/Accumulator  n_bits=FFTSize + 2*DataWidth + 2  overflow=Wrap  operation=Add  scale=1  explicit_period=off  period=1  rst=on  hasbypass=on  en=off  dbl_ovrd=off  show_param=off  gen_core=off  use_rpm=on
      settings: xl_area=[0, 0, 0, 0, 0, 0, 0]
  Accumulator1 : xbsIndex_r3/Accumulator  n_bits=FFTSize + 2*DataWidth + 2  overflow=Wrap  operation=Add  scale=1  explicit_period=off  period=1  rst=on  hasbypass=on  en=off  dbl_ovrd=off  show_param=off  gen_core=off  use_rpm=on
      settings: xl_area=[0, 0, 0, 0, 0, 0, 0]
  Constant : xbsIndex_r3/Constant  const=0  equ=P=C  arith_type=Unsigned  n_bits=FFTSize  bin_pt=0  opselect=C  inp2=PCIN>>17  opr=+  inp1=P  carry=CIN  iostate=0  explicit_period=off  period=1  dbl_ovrd=off
  Constant1 : xbsIndex_r3/Constant  const=2^(FFTSize+PFBSize)-1  equ=P=C  arith_type=Unsigned  n_bits=FFTSize+PFBSize  bin_pt=0  opselect=C  inp2=PCIN>>17  opr=+  inp1=P  carry=CIN  iostate=0  explicit_period=off  period=1  dbl_ovrd=off
  Convert : xbsIndex_r3/Convert  arith_type=Unsigned  n_bits=2*(DataWidth+1) + FFTSize  bin_pt=2*(DataWidth-1)  quantization=Truncate  overflow=Wrap  latency=0  explicit_period=off  period=1  dbl_ovrd=off  show_param=off  inserted_by_tool=off  pipeline=off
      settings: xl_area=[0, 0, 0, 0, 0, 0, 0]
  Convert1 : xbsIndex_r3/Convert  arith_type=Unsigned  n_bits=2*(DataWidth+1) + FFTSize  bin_pt=2*(DataWidth-1)  quantization=Truncate  overflow=Wrap  latency=0  explicit_period=off  period=1  dbl_ovrd=off  show_param=off  inserted_by_tool=off  pipeline=off
      settings: xl_area=[0, 0, 0, 0, 0, 0, 0]
  Convert2 : xbsIndex_r3/Convert  arith_type=Boolean  n_bits=FFTSize + 2*DataWidth + 1  bin_pt=2*DataWidth - 1  quantization=Truncate  overflow=Wrap  latency=0  explicit_period=off  period=1  dbl_ovrd=off  show_param=off  inserted_by_tool=off  pipeline=off
      settings: xl_area=[0, 0, 0, 0, 0, 0, 0]
  Counter : xbsIndex_r3/Counter  cnt_type=Free Running  n_bits=FFTSize+PFBSize  bin_pt=0  arith_type=Unsigned  start_count=0  cnt_to=Inf  cnt_by_val=1  operation=Up  explicit_period=off  period=1  load_pin=off  rst=on  en=off  dbl_ovrd=off  show_param=off  use_rpm=on  gen_core=off
      settings: xl_area=[0, 0, 0, 0, 0, 0, 0]
  Delay{,1..2,4} (4 alike) : xbsIndex_r3/Delay  latency=2  reg_retiming=off  explicit_period=off  period=1  en=off  accept_only_valid=off  init_zero=on  dbl_ovrd=off  show_param=off
      settings: xl_area=[0, 0, 0, 0, 0, 0, 0]
  Delay3 : xbsIndex_r3/Delay  Orientation=left  latency=1  reg_retiming=off  explicit_period=off  period=1  en=off  accept_only_valid=off  init_zero=on  dbl_ovrd=off  show_param=off
      settings: xl_area=[0, 0, 0, 0, 0, 0, 0]
  Delay5 : xbsIndex_r3/Delay  latency=1  reg_retiming=off  explicit_period=off  period=1  en=off  accept_only_valid=off  init_zero=on  dbl_ovrd=off  show_param=off
      settings: xl_area=[0, 0, 0, 0, 0, 0, 0]
  Expression : xbsIndex_r3/Expression  expression=a & ~b  precision=Full  arith_type=Unsigned  n_bits=8  bin_pt=2  align_bp=on  latency=0  explicit_period=off  period=1  en=off  dbl_ovrd=off  show_param=off
      settings: xl_area=[0, 0, 0, 0, 0, 0, 0]
  Gateway Out : xbsIndex_r3/Gateway Out  output_type=Double  nbits=8  bin_pt=6  arith_type=Boolean  quantization=Truncate  overflow=Wrap  hdl_port=off  timing_constraint=None  locs_specified=off  LOCs={}  needs_fixed_name=off  show_param=off
      settings: xl_area=[0, 0, 0, 0, 0, 0, 0]
  Gateway Out1 : xbsIndex_r3/Gateway Out  output_type=Double  nbits=8  bin_pt=6  arith_type=Boolean  quantization=Truncate  overflow=Wrap  hdl_port=off  timing_constraint=None  locs_specified=off  LOCs={}  needs_fixed_name=off  show_param=off
      settings: xl_area=[0, 0, 0, 0, 0, 0, 0]
  Gateway Out2 : xbsIndex_r3/Gateway Out  output_type=Double  nbits=8  bin_pt=6  arith_type=Boolean  quantization=Truncate  overflow=Wrap  hdl_port=off  timing_constraint=None  locs_specified=off  LOCs={}  needs_fixed_name=off  show_param=off
      settings: xl_area=[0, 0, 0, 0, 0, 0, 0]
  Logical : xbsIndex_r3/Logical  logical_function=XOR  inputs=2  precision=Full  arith_type=Unsigned  n_bits=8  bin_pt=2  align_bp=on  latency=0  explicit_period=off  period=1  en=off  dbl_ovrd=off  show_param=off
      settings: xl_area=[0, 0, 0, 0, 0, 0, 0]
  Logical1 : xbsIndex_r3/Logical  logical_function=AND  inputs=2  precision=Full  arith_type=Unsigned  n_bits=8  bin_pt=2  align_bp=on  latency=0  explicit_period=off  period=1  en=off  dbl_ovrd=off  show_param=off
      settings: xl_area=[0, 0, 0, 0, 0, 0, 0]
  Logical2 : xbsIndex_r3/Logical  logical_function=AND  inputs=2  precision=Full  arith_type=Unsigned  n_bits=8  bin_pt=2  align_bp=on  latency=0  explicit_period=off  period=1  en=off  dbl_ovrd=off  show_param=off
      settings: xl_area=[0, 0, 0, 0, 0, 0, 0]
  Register : xbsIndex_r3/Register  init=0  reg_only_valid=off  explicit_period=off  period=1  rst=off  en=on  out_en=off  dbl_ovrd=off  show_param=off
      settings: xl_area=[0, 0, 0, 0, 0, 0, 0]
  Register1 : xbsIndex_r3/Register  init=0  reg_only_valid=off  explicit_period=off  period=1  rst=off  en=on  out_en=off  dbl_ovrd=off  show_param=off
      settings: xl_area=[0, 0, 0, 0, 0, 0, 0]
  Register2 : xbsIndex_r3/Register  init=0  reg_only_valid=off  explicit_period=off  period=1  rst=on  en=on  out_en=off  dbl_ovrd=off  show_param=off
      settings: xl_area=[0, 0, 0, 0, 0, 0, 0]
  Register3 : xbsIndex_r3/Register  init=0  reg_only_valid=off  explicit_period=off  period=1  rst=on  en=on  out_en=off  dbl_ovrd=off  show_param=off
      settings: xl_area=[0, 0, 0, 0, 0, 0, 0]
  Register4 : xbsIndex_r3/Register  init=0  reg_only_valid=off  explicit_period=off  period=1  rst=on  en=on  out_en=off  dbl_ovrd=off  show_param=off
      settings: xl_area=[0, 0, 0, 0, 0, 0, 0]
  Register5 : xbsIndex_r3/Register  init=0  reg_only_valid=off  explicit_period=on  period=1  rst=on  en=on  out_en=off  dbl_ovrd=off  show_param=off
      settings: xl_area=[0, 0, 0, 0, 0, 0, 0]
  Relational : xbsIndex_r3/Relational  mode=a=b  latency=2  explicit_period=off  period=1  en=off  dbl_ovrd=off  show_param=off
      settings: xl_area=[0, 0, 0, 0, 0, 0, 0]
  Relational1 : xbsIndex_r3/Relational  mode=a!=b  latency=1  explicit_period=off  period=1  en=off  dbl_ovrd=off  show_param=off
      settings: xl_area=[0, 0, 0, 0, 0, 0, 0]
  Scope : Scope  NumInputPorts=3
      settings: YMin=-5~-5~-5  YMax=5~5~5  SaveName=ScopeData11
  Scope_Input : Subsystem
  Shift : xbsIndex_r3/Shift  shift_dir=Right  shift_bits=FFTSize  precision=User Defined  arith_type=Unsigned  n_bits=2*DataWidth + 1  bin_pt=2*(DataWidth - 1)  quantization=Truncate  overflow=Wrap  latency=1  explicit_period=off  period=1  en=off  dbl_ovrd=off  show_param=off
      settings: xl_area=[0, 0, 0, 0, 0, 0, 0]
  Shift1 : xbsIndex_r3/Shift  shift_dir=Right  shift_bits=FFTSize  precision=User Defined  arith_type=Unsigned  n_bits=2*DataWidth + 1  bin_pt=2*(DataWidth - 1)  quantization=Truncate  overflow=Wrap  latency=1  explicit_period=off  period=1  en=off  dbl_ovrd=off  show_param=off
      settings: xl_area=[0, 0, 0, 0, 0, 0, 0]
  Slice : xbsIndex_r3/Slice  mode=Lower Bit Location + Width  nbits=FFTSize  bit1=0  base1=MSB of Input  bit0=0  base0=LSB of Input  boolean_output=off  explicit_period=off  period=1  dbl_ovrd=off
  avgout1 : Outport
  avgout2 : Outport  Port=2
  valid : Outport  Port=3
  pout_sync : Outport  Port=4
  wires:
  Gateway Out2/1 -> Scope/3
  Gateway Out1/1 -> Scope/2
  Gateway Out/1 -> Scope/1
  Delay5/1 -> Register2/3, Register2/1
  Delay3/1 -> Relational1/1
  Constant1/1 -> Relational1/2
  Relational1/1 -> Logical2/2
  Logical2/1 -> Register2/2
  Slice/1 -> Relational/1
  Delay4/1 -> Delay5/1, Logical2/1
  Register2/1 -> Gateway Out2/1, Logical1/2
  Convert2/1 -> pout_sync/1
  Register4/1 -> Register3/1
  Expression/1 -> Convert2/1
  Register3/1 -> Register5/1, Logical/1, Expression/1
  Logical/1 -> Register5/3
  Register5/1 -> Logical/2, Expression/2
  Logical1/1 -> Gateway Out/1, Delay2/1
  Relational/1 -> Register3/3, Register4/3, Register4/1, Gateway Out1/1, Logical1/1, Accumulator/2, Register/2, Accumulator1/2, Register1/2
  pin1/1 -> Scope_Input/1(DataA), Convert/1
  pin2/1 -> Convert1/1
  Convert/1 -> Delay/1
  pin_sync/1 -> Register5/2, Register3/2, Register4/2, Delay4/1, Counter/1
  Counter/1 -> Delay3/1, Slice/1
  Constant/1 -> Relational/2
  Delay/1 -> Scope_Input/2(DataB), Accumulator/1
  Accumulator/1 -> Register/1
  Register/1 -> Scope_Input/3(DataC), Shift/1
  Shift/1 -> Scope_Input/4(Sync), avgout1/1
  Convert1/1 -> Delay1/1
  Delay1/1 -> Accumulator1/1
  Accumulator1/1 -> Register1/1
  Register1/1 -> Shift1/1
  Shift1/1 -> avgout2/1
  Delay2/1 -> valid/1
